simulink subsystem "Sub"  (R2023b)
settings: Solver=VariableStepAuto  StartTime=0.0  StopTime=10.0  RelTol=1e-3
libraries: frdmk64flib x1, dspstat3 x1
settings Model: Creator=haley  LastModifiedBy=haley

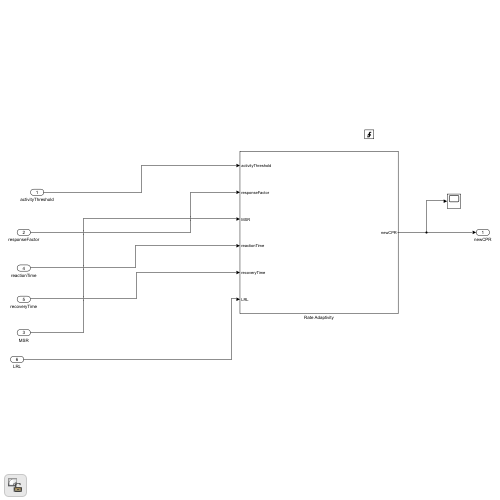
[thumbnail: Simulink's stored preview of the top-level diagram]
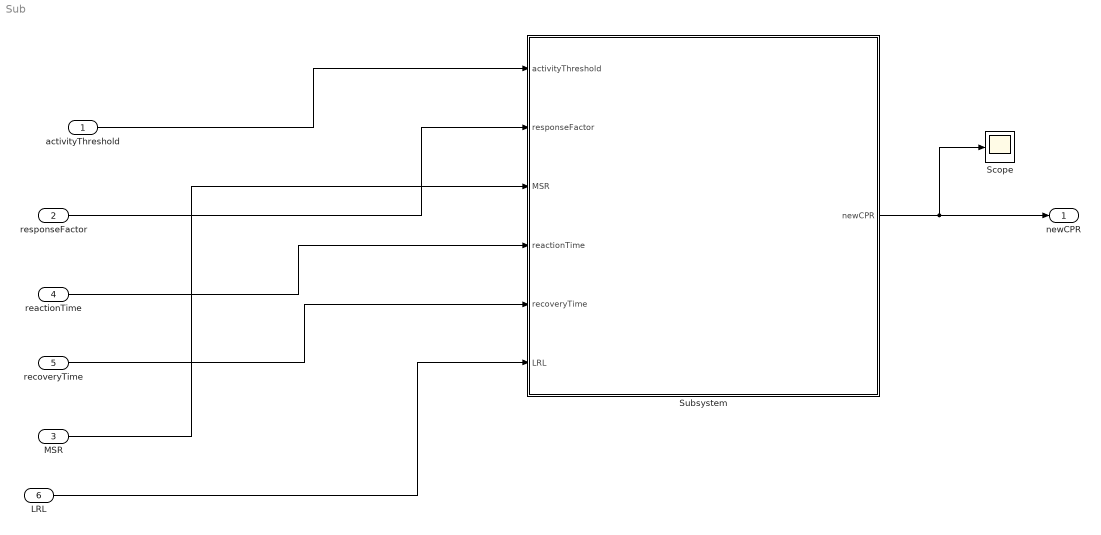
== system Sub ==
  activityThreshold : Inport
  responseFactor : Inport  Port=2
  MSR : Inport  Port=3
  reactionTime : Inport  Port=4
  recoveryTime : Inport  Port=5
  LRL : Inport  Port=6
  Scope : Scope
  Subsystem : Subsystem
  newCPR : Outport
  wires:
  Subsystem/1(newCPR) -> newCPR/1, Scope/1
  activityThreshold/1 -> Subsystem/1(activityThreshold)
  responseFactor/1 -> Subsystem/2(responseFactor)
  MSR/1 -> Subsystem/3(MSR)
  reactionTime/1 -> Subsystem/4(reactionTime)
  recoveryTime/1 -> Subsystem/5(recoveryTime)
  LRL/1 -> Subsystem/6(LRL)

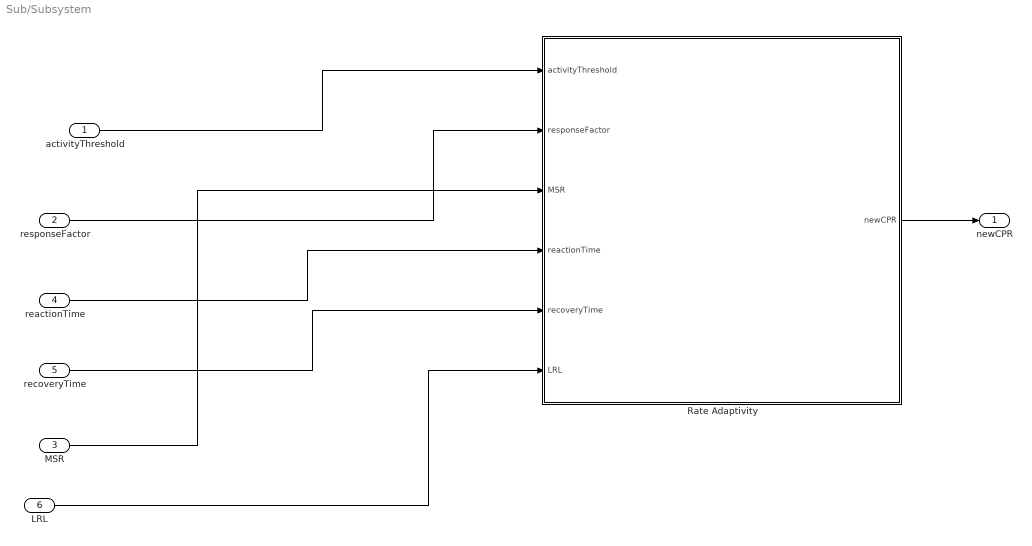
== system Sub/Subsystem ==
  activityThreshold : Inport
  responseFactor : Inport  Port=2
  MSR : Inport  Port=3
  reactionTime : Inport  Port=4
  recoveryTime : Inport  Port=5
  LRL : Inport  Port=6
  Rate Adaptivity : Subsystem
  newCPR : Outport
  wires:
  responseFactor/1 -> Rate Adaptivity/2(responseFactor)
  reactionTime/1 -> Rate Adaptivity/4(reactionTime)
  LRL/1 -> Rate Adaptivity/6(LRL)
  activityThreshold/1 -> Rate Adaptivity/1(activityThreshold)
  recoveryTime/1 -> Rate Adaptivity/5(recoveryTime)
  MSR/1 -> Rate Adaptivity/3(MSR)
  Rate Adaptivity/1(newCPR) -> newCPR/1

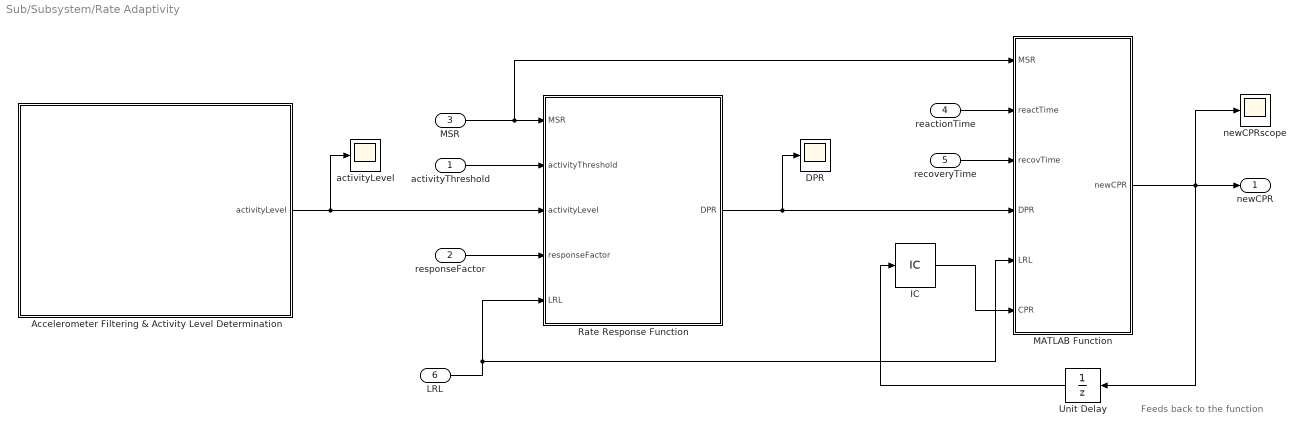
== system Sub/Subsystem/Rate Adaptivity ==
  note: Feeds back to the function
  activityThreshold : Inport
  responseFactor : Inport  Port=2
  MSR : Inport  Port=3
  reactionTime : Inport  Port=4
  recoveryTime : Inport  Port=5
  LRL : Inport  Port=6
  Accelerometer Filtering & Activity Level Determination : Subsystem
  DPR : Scope
  IC : InitialCondition  Value=60
  MATLAB Function : MATLAB Function  TreatAsAtomicUnit=on
  Rate Response Function : MATLAB Function  TreatAsAtomicUnit=on
  Unit Delay : UnitDelay  SampleTime=-1  HasFrameUpgradeWarning=on
  activityLevel : Scope
  newCPRscope : Scope
  newCPR : Outport
  wires:
  Accelerometer Filtering & Activity Level Determination/1(activityLevel) -> activityLevel/1, Rate Response Function/3(activityLevel)
  IC/1 -> MATLAB Function/6(CPR)
  Unit Delay/1 -> IC/1
  Rate Response Function/1(DPR) -> DPR/1, MATLAB Function/4(DPR)
  reactionTime/1 -> MATLAB Function/2(reactTime)
  MATLAB Function/1(newCPR) -> newCPRscope/1, newCPR/1, Unit Delay/1
  recoveryTime/1 -> MATLAB Function/3(recovTime)
  responseFactor/1 -> Rate Response Function/4(responseFactor)
  MSR/1 -> Rate Response Function/1(MSR), MATLAB Function/1(MSR)
  activityThreshold/1 -> Rate Response Function/2(activityThreshold)
  LRL/1 -> Rate Response Function/5(LRL), MATLAB Function/5(LRL)

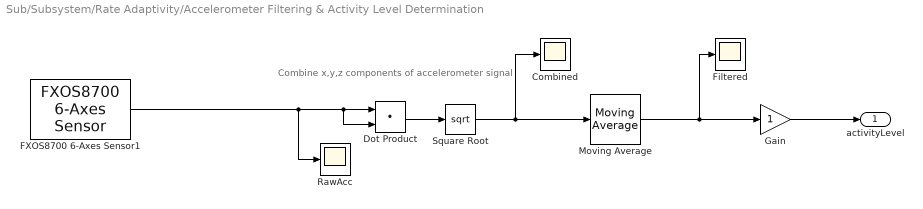
== system Sub/Subsystem/Rate Adaptivity/Accelerometer Filtering & Activity Level Determination ==
  note: Combine x,y,z components of accelerometer signal
  Combined : Scope
  Dot Product : DotProduct  OutDataTypeStr=Inherit: Inherit via internal rule
  FXOS8700 6-Axes Sensor1 : frdmk64flib/FXOS8700 6-Axes Sensor  Activesensor=Accelerometer only  ODR=800Hz  HybridODR=400Hz  Accelfullrange=-4g to +4g  SampleTime=-1
  Filtered : Scope
  Gain : Gain
  Moving Average : dspstat3/Moving Average  Method=Sliding window  ForgettingFactorPort=off  SpecifyWindowLength=on  WindowLength=4  OverlapLength=3  AllowArbitraryInputLength=off  ForgettingFactor=0.9  SimulateUsing=Code generation
  RawAcc : Scope
  Square Root : Sqrt
  activityLevel : Outport
  wires:
  FXOS8700 6-Axes Sensor1/1 -> RawAcc/1, Dot Product/2, Dot Product/1
  Gain/1 -> activityLevel/1
  Dot Product/1 -> Square Root/1
  Square Root/1 -> Combined/1, Moving Average/1
  Moving Average/1 -> Gain/1, Filtered/1

== matlab function Sub/Subsystem/Rate Adaptivity/MATLAB Function ==
  data: MSR input; newCPR output; reactTime input; recovTime input; DPR input; LRL input; CPR input
    function newCPR = timing(MSR, reactTime, recovTime, DPR, LRL, CPR)
if (CPR < DPR) && (CPR < MSR) % Increase Rate

    % Current Time based on Current Pace
    currTime = -log(1 - (LRL - CPR)/(LRL - MSR))*(reactTime/11 - 2/11);
    % Increase current time by 1ms
    currTime = currTime + 0.001;
    % New Pace Rate after 1ms increase
    newCPR = (1-exp(-11*currTime/(reactTime-2)))*(MSR-LRL) + LRL;

elseif (CPR > DPR) && (CPR > LRL) % Decrease Rate

    %Current Time based on Current Pace
    currTime = -log((LRL - CPR)/(LRL - MSR))*(recovTime/11 - 3/11);
    % Increase time by 1ms
    currTime = currTime + 0.001;
    %New Pace Rate after 1ms increase
    newCPR = (exp(-11*currTime/(recovTime-3)))*(MSR-LRL) + LRL;
      
else 
    newCPR = CPR; 

end
end

== matlab function Sub/Subsystem/Rate Adaptivity/Rate Response Function ==
  data: MSR input; activityThreshold input; DPR output; activityLevel input; responseFactor input; LRL input
function DPR  = fcn(MSR, activityThreshold, activityLevel, responseFactor, LRL)

% total range of change of acceleration 
ATMax = sqrt(4^2+4^2+4^2)-1; 

% since the accelerameter record the gravity (1g), 1g is removed to ensure when the pacemaker is static, there is no extra pacing 
activityThresholdLevels = {'V-Low', 'Low', 'Med-Low', 'Med', 'Med-High', 'High', 'V-High'}; %possible activity level string inputs

activityThresholdRange = [0.05*ATMax+1, 0.15*ATMax+1, 0.30*ATMax+1, 0.45*ATMax+1, 0.60*ATMax+1, 0.75*ATMax+1, 0.90*ATMax+1]; 
%take percentage of a maximum activity level, plus on to ensure the threshold is higher than defaul 1g (default acceleration reading

activityThresholdNum = activityThresholdRange(find(strcmp(activityThresholdLevels, char(activityThreshold)))); 
%map the string level of activity levels to a number value


if(activityLevel <= activityThresholdNum(1)) %doesn't meet the activity level threshold
    DPR = LRL;

elseif(activityLevel > activityThresholdNum(1) && activityLevel < sqrt(48))  % when the activity level is between threshold and max activity
    DPR = (1-exp((-(1/(sqrt(48)-activityLevel)*responseFactor*(activityLevel-activityThresholdNum(1))))))*(MSR-LRL)+LRL;

else
    DPR = MSR; %set to max sensor rate if activity level is greater than max activity

end
end
